simulink model "Model"  (R2023a)
settings: Solver=FixedStepAuto  StartTime=0.0  StopTime=4  FixedStep=0.0001  RelTol=1e-3
libraries: dspfdesign x2, spspowerguiLib x1
settings Model: SimulationMode=accelerator  Creator=04  LastModifiedBy=23688
settings SolverCC: AlgebraicLoopSolver=TrustRegion
settings DataIOCC: ReturnWorkspaceOutputs=off
settings DebuggingCC: UnconnectedInputMsg=warning  UnconnectedOutputMsg=warning  UnconnectedLineMsg=warning
settings ModelReferenceCC: EnableRefExpFcnMdlSchedulingChecks=on
settings RTWCC: DLArmComputeVersion=19.05

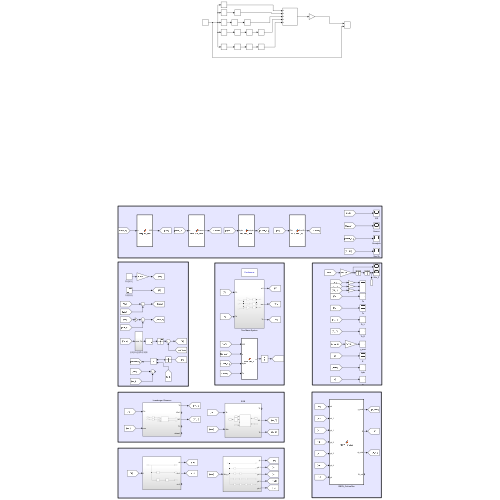
[thumbnail: Simulink's stored preview of the top-level diagram]
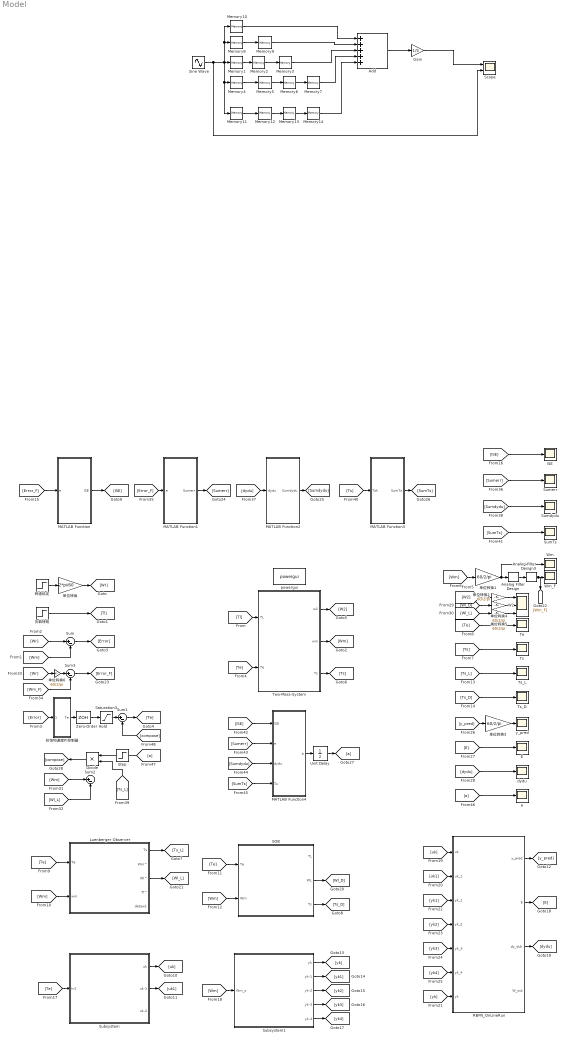
== system Model ==
  " Luenberger Observer" : Subsystem
  Add : Sum  Inputs=+++++
  Analog Filter Design : dspfdesign/Analog Filter Design  method=Butterworth  filttype=Bandstop  N=12  Wlo=700*2*pi  Whi=1300*2*pi  Rp=2  Rs=40
  Analog Filter Design3 : dspfdesign/Analog Filter Design  method=Butterworth  filttype=Bandstop  N=12  Wlo=900*2*pi  Whi=1100*2*pi  Rp=2  Rs=40
  Divide : Product  Inputs=**
  E : Scope
  Gain : Gain  Gain=1/5
  ISE : Scope
  MATLAB Function : MATLAB Function  TreatAsAtomicUnit=on
  MATLAB Function1 : MATLAB Function  TreatAsAtomicUnit=on
  MATLAB Function2 : MATLAB Function  TreatAsAtomicUnit=on
  MATLAB Function3 : MATLAB Function  TreatAsAtomicUnit=on
  MATLAB Function4 : MATLAB Function  TreatAsAtomicUnit=on
  Memory{1..14} (14 alike) : Memory  InitialCondition=0.001
  RBFN_OnLineRun : MATLAB Function  TreatAsAtomicUnit=on
  SOB : Subsystem
  Saturation3 : Saturate  UpperLimit=2.39*3  LowerLimit=-2.39*3
  Scope : Scope  NumInputPorts=2
  Sine Wave : Sin  Frequency=1000*2*pi  SampleTime=0
  Step : Step  Time=2  After=0.5  SampleTime=0
  Subsystem : Subsystem
  Subsystem1 : Subsystem
  Sum{,1..3} (4 alike) : Sum  Inputs=|+-
  SumTs : Scope
  Sumdydu : Scope
  Sumerr : Scope
  Te : Scope
  Ts : Scope
  Ts_D : Scope
  Ts_L : Scope
  Two-Mass-System : Subsystem
  Unit Delay : UnitDelay  SampleTime=-1  HasFrameUpgradeWarning=on
  W2 : Scope  NumInputPorts=3
  Wm : Scope
  Wm_F : Scope
  Zero-Order Hold : ZeroOrderHold  SampleTime=0.0005
  a : Scope
  dydu : Scope
  powergui : spspowerguiLib/powergui  Priority=1  SimulationMode=Continuous  SampleTime=50e-6  frequency=60  Iterations=50  frequencyindice=60  Pbase=100e6  ErrMax=1e-4  UnitsV=kV  UnitsW=MW  buscounter=0  FunctionMessages=off  echomessages=off  EnableUseOfTLC=off  CurrentSourceSwitches=off  DisableSnubberDevices=off  DisableRonSwitches=off  DisableVfSwitches=off  DisplayEquations=off  AutomaticDiscreteSolvers=off  SolverType=Tustin/Backward Euler (TBE)  Interpol=off  ExternalGateDelay=off  methode=off  Ts=100  x0status=blocks  SPID=on  SwTol=0  HookPort=off  NonlinearTolerance=1e-4  nMaxIteration=100  ContinueOnMaxIteration=off  RestoreLinks=warning  ResistiveCurrentMeasurement=off  Frange=[0:2:500]  Ylog=off  Xlog=on  ShowGrid=off  save=off  variable=ZData  structure=0  ZoomFFT=off  StartTime=0.0  cycles=1  DisplayStyle=1  fundamental=60  FreqAxis=off  MaxFrequency=1000  frequencyindicesteady=1  RmsSteady=1  display=off
  y_pred : Scope
  单位转换 : Gain  Gain=2*pi/60
  单位转换{1..6} (6 alike) : Gain  Gain=60/2/pi
  抗饱和速度PI控制器 : Subsystem
  负载转矩 : Step  Time=0  After=0  SampleTime=0
  转速给定 : Step  Time=0.1  After=1000  SampleTime=0
  wires:
  Memory1/1 -> Memory2/1
  Memory2/1 -> Memory3/1
  Memory4/1 -> Memory5/1
  Memory5/1 -> Memory6/1
  Memory6/1 -> Memory7/1
  Memory8/1 -> Memory9/1
  Memory10/1 -> Add/1
  Memory9/1 -> Add/2
  Memory3/1 -> Add/3
  Memory7/1 -> Add/4
  Memory14/1 -> Add/5
  Memory13/1 -> Memory14/1
  Memory12/1 -> Memory13/1
  Memory11/1 -> Memory12/1
  Sine Wave/1 -> Scope/2, Memory10/1, Memory8/1, Memory11/1, Memory4/1, Memory1/1
  Add/1 -> Gain/1
  Gain/1 -> Scope/1
  转速给定/1 -> 单位转换/1
  负载转矩/1 -> [Tl]
  [Tl] -> Two-Mass-System/1(TL)
  Two-Mass-System/2(wm) -> [Wm]
  [Wr] -> Sum/1
  [Wm] -> Sum/2
  Sum/1 -> [Error]
  [Error] -> 抗饱和速度PI控制器/1(error)
  Two-Mass-System/1(w2) -> [W2]
  Two-Mass-System/3(Ts) -> [Ts]
  [Ts] -> Ts/1
  [Te] -> Te/1
  单位转换/1 -> [Wr]
  [Wm] -> 单位转换1/1
  [Te] -> " Luenberger Observer"/1(Te)
  [Wm] -> " Luenberger Observer"/2(wm)
  [Te] -> SOB/1(Te)
  [Wm] -> SOB/2(Wm)
  " Luenberger Observer"/1(Ts) -> [Ts_L]
  SOB/3(Ts) -> [Ts_D]
  [Ts_L] -> Ts_L/1
  [Ts_D] -> Ts_D/1
  [W2] -> 单位转换2/1
  单位转换2/1 -> W2/1
  [Error_F] -> MATLAB Function/1(e)
  MATLAB Function/1(ISE) -> [ISE]
  [Te] -> Subsystem/1(In1)
  Subsystem/1(uk) -> [uk]
  Subsystem/2(uk-1) -> [uk1]
  [Wm] -> Subsystem1/1(Wm_o)
  Subsystem1/1(yk) -> [yk]
  Subsystem1/2(yk-1) -> [yk1]
  Subsystem1/3(yk-2) -> [yk2]
  Subsystem1/4(yk-3) -> [yk3]
  Subsystem1/5(yk-4) -> [yk4]
  [uk] -> RBFN_OnLineRun/1(uk)
  [uk1] -> RBFN_OnLineRun/2(uk_1)
  [yk] -> RBFN_OnLineRun/7(yk)
  [yk1] -> RBFN_OnLineRun/3(yk_1)
  [yk2] -> RBFN_OnLineRun/4(yk_2)
  [yk3] -> RBFN_OnLineRun/5(yk_3)
  [yk4] -> RBFN_OnLineRun/6(yk_4)
  RBFN_OnLineRun/1(y_pred) -> [y_pred]
  RBFN_OnLineRun/2(E) -> [E]
  RBFN_OnLineRun/3(dy_duk) -> [dydu]
  [E] -> E/1
  [dydu] -> dydu/1
  [y_pred] -> 单位转换3/1
  单位转换3/1 -> y_pred/1
  Sum1/1 -> [Te]
  SOB/2(WL) -> [Wl_D]
  " Luenberger Observer"/3(Wl^) -> [Wl_L]
  单位转换4/1 -> W2/2
  [Wl_D] -> 单位转换4/1
  单位转换5/1 -> W2/3
  [Wl_L] -> 单位转换5/1
  [Wm] -> Sum2/1
  [Wl_L] -> Sum2/2
  Analog Filter Design/1 -> Analog Filter Design3/1
  Analog Filter Design3/1 -> [Wm_F], Wm_F/1
  单位转换1/1 -> Wm/1, Analog Filter Design/1
  [Wr] -> 单位转换6/1
  单位转换6/1 -> Sum3/1
  [Wm_F] -> Sum3/2
  Sum3/1 -> [Error_F]
  [Error_F] -> MATLAB Function1/1(e)
  MATLAB Function1/1(Sumerr) -> [Sumerr]
  [ISE] -> ISE/1
  [Sumerr] -> Sumerr/1
  [dydu] -> MATLAB Function2/1(dydu)
  MATLAB Function2/1(Sumdydu) -> [Sumdydu]
  [Sumdydu] -> Sumdydu/1
  [Ts] -> MATLAB Function3/1(Tsk)
  MATLAB Function3/1(SumTs) -> [SumTs]
  [SumTs] -> SumTs/1
  [ISE] -> MATLAB Function4/1(ISE)
  [Sumerr] -> MATLAB Function4/2(e)
  [Sumdydu] -> MATLAB Function4/3(dydu)
  [SumTs] -> MATLAB Function4/4(Ts)
  MATLAB Function4/1(a) -> Unit Delay/1
  [a] -> a/1
  Unit Delay/1 -> [a]
  Divide/1 -> [compose]
  [compose] -> Sum1/2
  [Te] -> Two-Mass-System/2(Te)
  [Ts_L] -> Divide/2
  Saturation3/1 -> Sum1/1
  抗饱和速度PI控制器/1(Te) -> Zero-Order Hold/1
  Zero-Order Hold/1 -> Saturation3/1
  [a] -> Divide/1

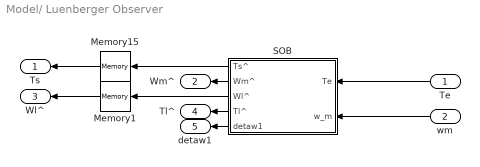
== system Model/ Luenberger Observer ==
  Te : Inport
  wm : Inport  Port=2
  Memory1 : Memory
  Memory15 : Memory
  SOB : Subsystem
  Ts : Outport
  Wm^ : Outport  Port=2
  Wl^ : Outport  Port=3
  Tl^ : Outport  Port=4
  detaw1 : Outport  Port=5
  wires:
  SOB/4(Tl^) -> Tl^/1
  SOB/1(Ts^) -> Memory15/1
  Memory15/1 -> Ts/1
  wm/1 -> SOB/2(w_m)
  SOB/2(Wm^) -> Wm^/1
  Te/1 -> SOB/1(Te)
  SOB/5(detaw1) -> detaw1/1
  Memory1/1 -> Wl^/1
  SOB/3(Wl^) -> Memory1/1

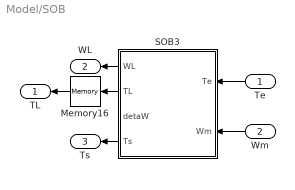
== system Model/SOB ==
  Te : Inport
  Wm : Inport  Port=2
  Memory16 : Memory
  SOB3 : Subsystem
  TL : Outport
  WL : Outport  Port=2
  Ts : Outport  Port=3
  wires:
  SOB3/1(WL) -> WL/1
  SOB3/4(Ts) -> Ts/1
  Wm/1 -> SOB3/2(Wm)
  Te/1 -> SOB3/1(Te)
  SOB3/2(TL) -> Memory16/1
  Memory16/1 -> TL/1

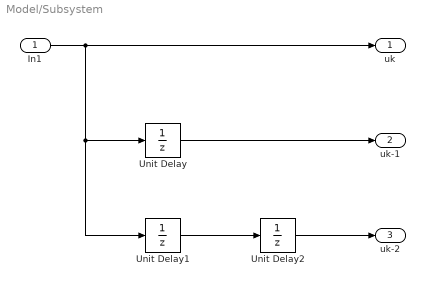
== system Model/Subsystem ==
  In1 : Inport
  Unit Delay : UnitDelay  SampleTime=-1  HasFrameUpgradeWarning=on
  Unit Delay1 : UnitDelay  SampleTime=-1  HasFrameUpgradeWarning=on
  Unit Delay2 : UnitDelay  SampleTime=-1  HasFrameUpgradeWarning=on
  uk : Outport
  uk-1 : Outport  Port=2
  uk-2 : Outport  Port=3
  wires:
  Unit Delay1/1 -> Unit Delay2/1
  Unit Delay/1 -> uk-1/1
  Unit Delay2/1 -> uk-2/1
  In1/1 -> Unit Delay1/1, Unit Delay/1, uk/1

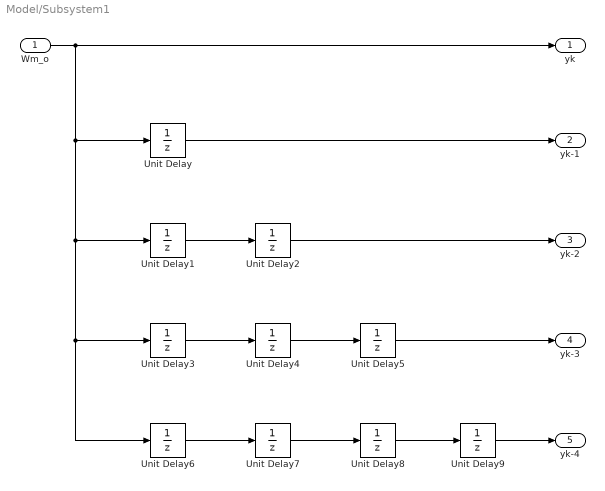
== system Model/Subsystem1 ==
  Wm_o : Inport
  Unit Delay{,1..9} (10 alike) : UnitDelay  SampleTime=-1  HasFrameUpgradeWarning=on
  yk : Outport
  yk-1 : Outport  Port=2
  yk-2 : Outport  Port=3
  yk-3 : Outport  Port=4
  yk-4 : Outport  Port=5
  wires:
  Unit Delay5/1 -> yk-3/1
  Unit Delay4/1 -> Unit Delay5/1
  Unit Delay2/1 -> yk-2/1
  Unit Delay8/1 -> Unit Delay9/1
  Unit Delay7/1 -> Unit Delay8/1
  Unit Delay6/1 -> Unit Delay7/1
  Unit Delay9/1 -> yk-4/1
  Unit Delay3/1 -> Unit Delay4/1
  Unit Delay/1 -> yk-1/1
  Wm_o/1 -> Unit Delay3/1, Unit Delay6/1, Unit Delay1/1, Unit Delay/1, yk/1
  Unit Delay1/1 -> Unit Delay2/1

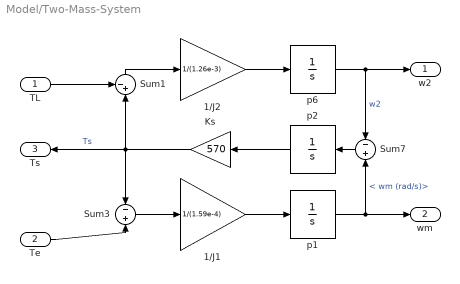
== system Model/Two-Mass-System ==
  TL : Inport
  Te : Inport  Port=2
  1/J1 : Gain  Gain=1/(1.59e-4)
  1/J2 : Gain  Gain=1/(1.26e-3)
  Ks : Gain  Gain=570
  Sum1 : Sum  Inputs=-+|
  Sum3 : Sum  Inputs=-+
  Sum7 : Sum  Inputs=-+
  p1 : TransferFcn  Denominator=[1 0]
  p2 : TransferFcn  Denominator=[1 0]
  p6 : TransferFcn  Denominator=[1 0]
  w2 : Outport
  wm : Outport  Port=2
  Ts : Outport  Port=3
  wires:
  Sum3/1 -> 1/J1/1
  1/J1/1 -> p1/1
  p1/1 -> wm/1, Sum7/2  "< wm (rad/s)>"
  p6/1 -> Sum7/1, w2/1  "w2"
  Sum7/1 -> p2/1
  Sum1/1 -> 1/J2/1
  Ks/1 -> Ts/1, Sum1/2, Sum3/1  "Ts"
  p2/1 -> Ks/1
  1/J2/1 -> p6/1
  TL/1 -> Sum1/1
  Te/1 -> Sum3/2

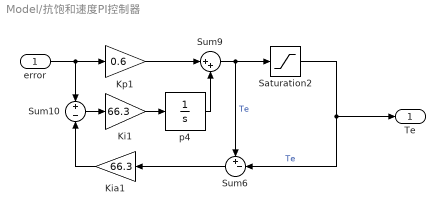
== system Model/抗饱和速度PI控制器 ==
  error : Inport
  Ki1 : Gain  Gain=66.3
  Kia1 : Gain  Gain=66.3
  Kp1 : Gain  Gain=0.6
  Saturation2 : Saturate  UpperLimit=2.39*3  LowerLimit=-2.39*3
  Sum10 : Sum  Inputs=+|-
  Sum6 : Sum  Inputs=+-|
  Sum9 : Sum  Inputs=|++
  p4 : TransferFcn  Denominator=[1 0]
  Te : Outport
  wires:
  Kia1/1 -> Sum10/2
  Sum6/1 -> Kia1/1
  Sum10/1 -> Ki1/1
  Kp1/1 -> Sum9/1
  Saturation2/1 -> Te/1, Sum6/2  "Te"
  Sum9/1 -> Sum6/1, Saturation2/1  "Te"
  p4/1 -> Sum9/2
  Ki1/1 -> p4/1
  error/1 -> Kp1/1, Sum10/1

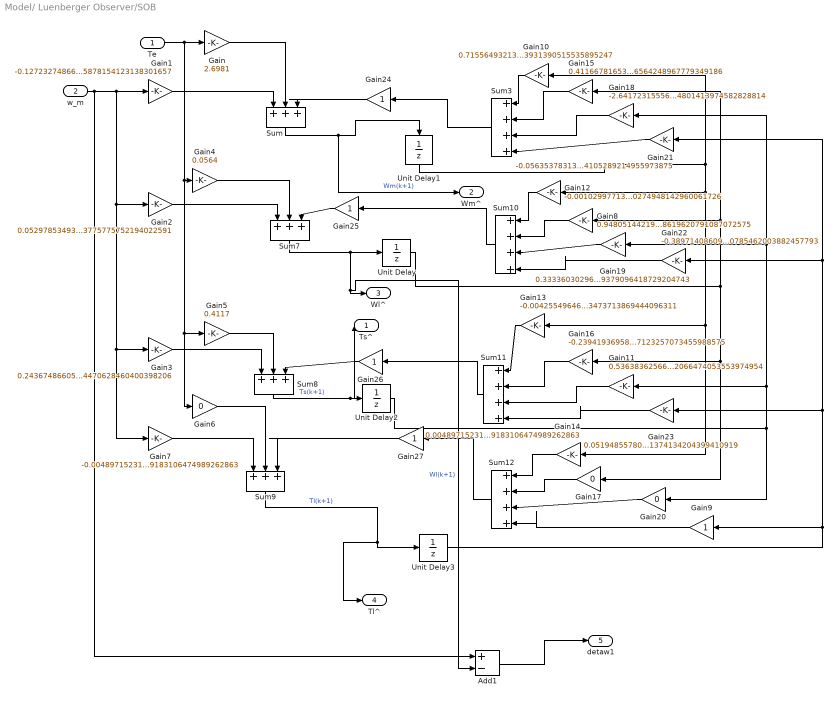
== system Model/ Luenberger Observer/SOB ==
  Te : Inport
  w_m : Inport  Port=2
  Add1 : Sum  Inputs=+-
  Gain : Gain  Gain=2.6981
  Gain1 : Gain  Gain=-0.12723274866755878154123138301657
  Gain10 : Gain  Gain=0.7155649321343931390515535895247
  Gain11 : Gain  Gain=0.53638362566622066474053553974954
  Gain12 : Gain  Gain=-0.0010299771306700274948142960061726
  Gain13 : Gain  Gain=-0.004255496467973473713869444096311
  Gain14 : Gain  Gain=0.0048971523131869183106474989262863
  Gain15 : Gain  Gain=0.41166781653316564248967779349186
  Gain16 : Gain  Gain=-0.23941936958917123257073455988575
  Gain17 : Gain  Gain=0
  Gain18 : Gain  Gain=-2.6417231555684801413974582828814
  Gain19 : Gain  Gain=0.33336030296459379096418729204743
  Gain2 : Gain  Gain=0.052978534931283775775752194022591
  Gain20 : Gain  Gain=0
  Gain21 : Gain  Gain=-0.056353783132214105289214955973875
  Gain22 : Gain  Gain=-0.38971408609680785462003882457793
  Gain23 : Gain  Gain=0.05194855780061374134204399410919
  Gain{9,24..27} (5 alike) : Gain
  Gain3 : Gain  Gain=0.24367486605714470628460400398206
  Gain4 : Gain  Gain=0.0564
  Gain5 : Gain  Gain=0.4117
  Gain6 : Gain  Gain=0
  Gain7 : Gain  Gain=-0.0048971523131869183106474989262863
  Gain8 : Gain  Gain=0.94805144219938619620791087072575
  Sum{,7..9} (4 alike) : Sum  Inputs=+++|
  Sum{3,10..12} (4 alike) : Sum  Inputs=++++|
  Unit Delay{,1..3} (4 alike) : UnitDelay  SampleTime=-1
  Ts^ : Outport
  Wm^ : Outport  Port=2
  Wl^ : Outport  Port=3
  Tl^ : Outport  Port=4
  detaw1 : Outport  Port=5
  wires:
  Te/1 -> Gain5/1, Gain6/1, Gain4/1, Gain/1
  Gain/1 -> Sum/2
  Gain1/1 -> Sum/1
  Gain4/1 -> Sum7/2
  Gain2/1 -> Sum7/1
  Gain5/1 -> Sum8/2
  Gain3/1 -> Sum8/1
  Gain6/1 -> Sum9/2
  Gain7/1 -> Sum9/1
  Sum/1 -> Unit Delay1/1, Wm^/1  "Wm(k+1)"
  Sum7/1 -> Add1/2, Wl^/1, Unit Delay/1  "Wl(k+1)"
  Sum8/1 -> Ts^/1, Unit Delay2/1  "Ts(k+1)"
  Sum9/1 -> Tl^/1, Unit Delay3/1  "Tl(k+1)"
  Sum12/1 -> Gain27/1
  Gain10/1 -> Sum3/1
  Gain11/1 -> Sum11/3
  Gain9/1 -> Sum12/4
  Gain12/1 -> Sum10/1
  Gain13/1 -> Sum11/1
  Gain14/1 -> Sum12/1
  Gain17/1 -> Sum12/2
  Gain19/1 -> Sum10/3
  Unit Delay1/1 -> Gain14/1, Gain13/1, Gain12/1, Gain10/1
  Unit Delay/1 -> Gain8/1, Gain15/1, Gain17/1, Gain16/1
  Unit Delay2/1 -> Gain11/1, Gain18/1, Gain19/1, Gain20/1
  Unit Delay3/1 -> Gain21/1, Gain22/1, Gain23/1, Gain9/1
  Gain25/1 -> Sum7/3
  Gain26/1 -> Sum8/3
  Sum3/1 -> Gain24/1
  Gain24/1 -> Sum/3
  Gain15/1 -> Sum3/2
  Gain18/1 -> Sum3/3
  Gain21/1 -> Sum3/4
  Sum10/1 -> Gain25/1
  Gain8/1 -> Sum10/2
  Sum11/1 -> Gain26/1
  Gain16/1 -> Sum11/2
  Gain23/1 -> Sum11/4
  Gain27/1 -> Sum9/3
  Gain20/1 -> Sum12/3
  Gain22/1 -> Sum10/4
  Add1/1 -> detaw1/1
  w_m/1 -> Add1/1, Gain3/1, Gain7/1, Gain2/1, Gain1/1

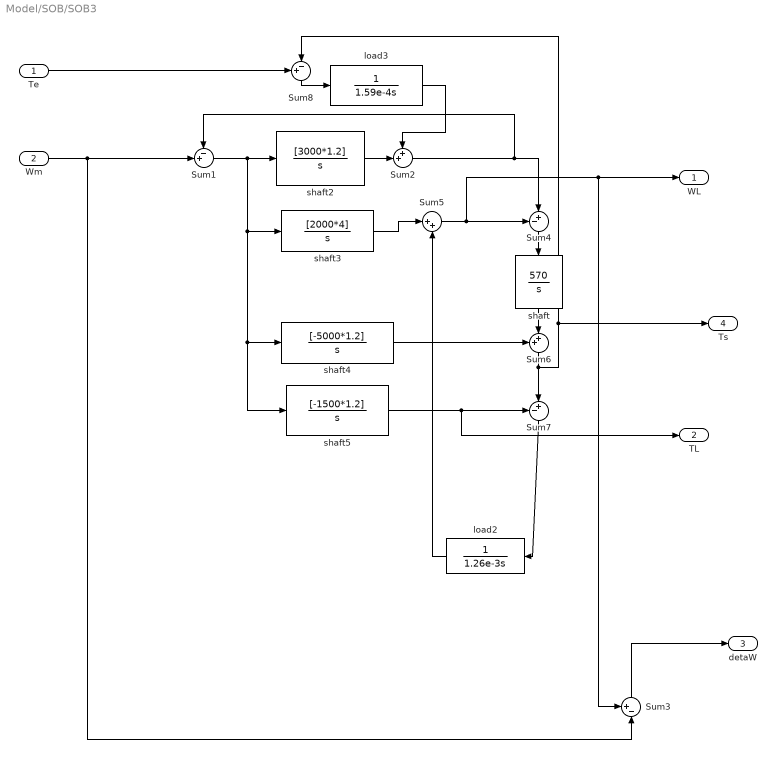
== system Model/SOB/SOB3 ==
  Te : Inport
  Wm : Inport  Port=2
  Sum1 : Sum  Inputs=-+|
  Sum2 : Sum  Inputs=++|
  Sum3 : Sum  Inputs=+-|
  Sum4 : Sum  Inputs=-+|
  Sum5 : Sum  Inputs=|++
  Sum6 : Sum  Inputs=++|
  Sum7 : Sum  Inputs=-+|
  Sum8 : Sum  Inputs=+-|
  load2 : TransferFcn  Denominator=[1.26e-3 0]
  load3 : TransferFcn  Denominator=[1.59e-4 0]
  shaft : TransferFcn  Numerator=[570]  Denominator=[1 0]
  shaft2 : TransferFcn  Numerator=[3000*1.2]  Denominator=[1 0]
  shaft3 : TransferFcn  Numerator=[2000*4]  Denominator=[1 0]
  shaft4 : TransferFcn  Numerator=[-5000*1.2]  Denominator=[1 0]
  shaft5 : TransferFcn  Numerator=[-1500*1.2]  Denominator=[1 0]
  WL : Outport  VectorParamsAs1DForOutWhenUnconnected=off
  TL : Outport  Port=2  VectorParamsAs1DForOutWhenUnconnected=off
  detaW : Outport  Port=3  VectorParamsAs1DForOutWhenUnconnected=off
  Ts : Outport  Port=4  VectorParamsAs1DForOutWhenUnconnected=off
  wires:
  Wm/1 -> Sum1/2, Sum3/2
  Te/1 -> Sum8/1
  load3/1 -> Sum2/1
  Sum8/1 -> load3/1
  load2/1 -> Sum5/2
  Sum7/1 -> load2/1
  Sum6/1 -> Sum7/2, Ts/1, Sum8/2
  shaft5/1 -> TL/1, Sum7/1
  shaft/1 -> Sum6/2
  shaft4/1 -> Sum6/1
  Sum4/1 -> shaft/1
  Sum5/1 -> WL/1, Sum3/1, Sum4/1
  shaft3/1 -> Sum5/1
  Sum2/1 -> Sum4/2, Sum1/1
  shaft2/1 -> Sum2/2
  Sum1/1 -> shaft5/1, shaft4/1, shaft3/1, shaft2/1
  Sum3/1 -> detaW/1

== matlab function Model/RBFN_OnLineRun ==
  settings: updateMethod=DISCRETE  sampleTime=0.0001
  data: y_pred output; uk input; E output; uk_1 input; yk_1 input; yk_2 input; yk_3 input; yk_4 input; yk input; dy_duk output; W_out output
function [y_pred, E, dy_duk,W_out]  = RBFN_OnLine(uk, uk_1, yk_1, yk_2, yk_3, yk_4, yk)

%6个输入，包含当前、过去输入与过去输出
u = [uk; uk_1; yk_1; yk_2; yk_3; yk_4]; % [6 x 1]

%RBFN参数定义与初始化
persistent centers sigma W learning

if isempty(centers)

    %从文件中加载预训练的参数，注意文件名
    data = load('RBFN_parameters2.mat');
    centers = data.centers;
    sigma = data.sigma;
    W = data.W_init;
    learning = true;

end

K = 36; % 神经元数量
H = zeros(K, 1);

% 计算偏导数
delta = zeros(K, 1); 

for j = 1:K
    % 计算第 j 个 RBF 神经元的输出
    distance = norm(u - centers(j, :)'); 
    H(j) = exp(- (distance^2) / (2 * sigma^2));

    % c_{j1} 是 centers 矩阵的第 j 行，第1个元素，也就是uk所具体对应的中心值，因为有36个神经元，所以对应36个值
    delta(j) = uk - centers(j, 1);
end

% 计算网络的预测输出
y_pred = W' * H;

% 计算预测误差
e = yk - y_pred;
E = e;

% 学习率设置
eta_W = 0.10;    
eta_c = 0.008;    
eta_sigma = 0.005; 

epsilon = 0.01; % 误差阈值

% 判断是否需要更新参数，误差没有达到要求就更新
if learning
    W = W + eta_W * e * H;

    for j = 1:K
        centers(j, :) = centers(j, :) + ...
            eta_c * e * W(j) * H(j) * (u' - centers(j, :)) / sigma^2;
    end

    delta_sigma = 0;

    for j = 1:K
        delta_sigma = delta_sigma + ...
            e * W(j) * H(j) * (norm(u - centers(j, :)')^2) / sigma^3;
    end
    
    sigma = sigma + eta_sigma * delta_sigma / K;
end

% 收敛条件判断
if abs(e) < epsilon
    % 误差小于阈值，停止参数更新
    learning = false;
else
    % 误差大于阈值，继续参数更新
    learning = true;
end

% 计算网络输出 y 关于当前输入 u_k 的偏导数

% 推导公式：
% dy/du_k = - (1 / sigma^2) * sum_{j=1}^K [ W_j * H_j * (u_k - c_{j1}) ]

% 计算偏导数
dy_duk = - (1 / sigma^2) * sum(W .* H .* delta);
W_out = W;


end

== matlab function Model/MATLAB Function ==
  settings: updateMethod=DISCRETE  sampleTime=0.0001
  data: e input; ISE output
function ISE = compute_ISE(e)

persistent T time M SumErr SumOut N SumAvg SumISE

if isempty(T)
    T = 0.0001;
    time = 0;
    SumErr = 0;
    SumOut = 0;
    SumAvg = 0;
    SumISE = 0;
    M = 0;
    N = 0;
end

if (time >= 2)

    SumErr = SumErr + e^2 * T;
    M = M + 1;

    if (M == 50)
        SumISE = SumErr;
        SumOut = SumOut + SumISE;
        M = 0;
        SumErr = 0;
        N = N + 1;
        
        if (N == 10)
            SumAvg = SumOut / 10;
            N = 0;
            SumOut = 0;
        end
    end

end

time = time + T;

ISE = SumAvg;

end

== matlab function Model/MATLAB Function1 ==
  settings: updateMethod=DISCRETE  sampleTime=0.0001
  data: e input; Sumerr output
function Sumerr = calculate_error(e)

persistent T time Err M ErrOut N ErrAvg

if isempty(T)
    T = 0.0001;
    time = 0;
    Err = 0;
    M = 0;
    ErrOut = 0;
    N = 0;
    ErrAvg = 0;
end

if (time > 2)

    Err = Err + e;
    M = M + 1;

    if (M == 50)
        ErrOut = ErrOut + Err;
        N = N + 1;
        Err = 0;
        M = 0;

        if (N == 10)
            ErrAvg = ErrOut / 10;
            N = 0;
            ErrOut = 0;
        end

    end

end

time = time + T;

Sumerr = ErrAvg;

end

== matlab function Model/MATLAB Function2 ==
  settings: updateMethod=DISCRETE  sampleTime=0.0001
  data: dydu input; Sumdydu output
function Sumdydu = calculate_dydu(dydu)

persistent T time dydu_sum M dyduOut N dyduAvg

if isempty(T)
    T = 0.0001;
    time = 0;
    dydu_sum = 0;
    M = 0;
    dyduOut = 0;
    N = 0;
    dyduAvg = 0;
end

if (time > 2)

    dydu_sum = dydu_sum + dydu;
    M = M + 1;

    if (M == 50)
        dyduOut = dyduOut + dydu_sum;
        N = N + 1;
        dydu_sum = 0;
        M = 0;

        if (N == 10)
            dyduAvg = dyduOut / 10;
            N = 0;
            dyduOut = 0;
        end

    end

end

time = time + T;

Sumdydu = dyduAvg;

end

== matlab function Model/MATLAB Function3 ==
  settings: updateMethod=DISCRETE  sampleTime=0.0001
  data: Tsk input; SumTs output
function SumTs = calculate_Ts(Tsk)

persistent T time Ts_sum M TsOut N TsAvg

if isempty(T)
    T = 0.0001;
    time = 0;
    Ts_sum = 0;
    M = 0;
    TsOut = 0;
    N = 0;
    TsAvg = 0;
end

if (time > 2)

    Ts_sum = Ts_sum + Tsk;
    M = M + 1;

    if (M == 100)
        TsOut = TsOut + Ts_sum;
        N = N + 1;
        Ts_sum = 0;
        M = 0;

        if (N == 10)
            TsAvg = TsOut / 10;
            N = 0;
            TsOut = 0;
        end

    end

end

time = time + T;

SumTs = TsAvg;

end

== matlab function Model/MATLAB Function4 ==
  settings: updateMethod=DISCRETE  sampleTime=0.0001
  data: ISE input; a output; e input; dydu input; Ts input
function a = calculate_a(ISE,e,dydu,Ts)
persistent T time a_now a_old eta_a

if isempty(T)
    T = 0.0001;
    time = 0;
    a_old = 0;
    a_now = 0.0;
    eta_a = 0.85;
end

if (time > 2.1)
    if (ISE > 0.1)
        a_now = a_old - eta_a * 2 * ISE * e * dydu * Ts * 1; %一般是乘以0.0001，也就是T，这个值很小，会导致收敛速度很慢

        if (a_now > 1.2)
            a_now = 0.9;
        end

        if (a_now < 0)
            a_now = 0;
        end
    else
        a_now = a_old;
    end
end

time = time + T;

a = a_now;
a_old = a_now;

end
